simulink model "DA42_Validations"  (Simulink 7.5)
settings: Solver=ode3  StartTime=0.0  StopTime=fdata(end,1)  FixedStep=0.02  RelTol=1e-3
undefined symbols (not defined in the file or in its folder): BHP_A, BHP_B, CP_norm, elebias, fdata, initalt, initbank, initeast, inithead, initnorth, initp, initpitch, initq, initr, initu, initv, initw, mapbias, Pr_Alt, PropEff_norm
libraries: simulink_extras x4, aerolibatmos2 x2
(part 2 of 2)

== system DA42_Validations/DA42/Linear Accelerations and Moments/Cross Prod Moment due to Aero ==
  Vec 1 : Inport
  Vec 2 : Inport  Port=2
  Demux : Demux  Outputs=3
  Demux1 : Demux  Outputs=3
  J axis : Fcn  Expr=u[4]*u[3] - u[6]*u[1]
  Mux : Mux  Inputs=6
  Mux1 : Mux  Inputs=3
  i axis : Fcn  Expr=u[6]*u[2] - u[5]*u[3]
  k axis : Fcn  Expr=u[5]*u[1] - u[4]*u[2]
  X Prod : Outport
  wires:
  Mux1/1 -> X Prod/1
  k axis/1 -> Mux1/3
  i axis/1 -> Mux1/1
  J axis/1 -> Mux1/2
  Mux/1 -> k axis/1, J axis/1, i axis/1
  Demux/2 -> Mux/2
  Demux/3 -> Mux/3
  Demux1/1 -> Mux/4
  Demux1/2 -> Mux/5
  Demux1/3 -> Mux/6
  Demux/1 -> Mux/1
  Vec 1/1 -> Demux/1
  Vec 2/1 -> Demux1/1

== system DA42_Validations/DA42/Linear Accelerations and Moments/Thrust Components ==
  Feng : Inport
  Bus Selector : BusSelector  OutputSignals=L_Thrust,R_Thrust
  Sum : Sum  Inputs=|++
  X Percent : Gain  Gain=0.9669
  Y Percent : Gain  Gain=0
  Z Percent : Gain  Gain=-0.03310
  X% : Outport
  Y% : Outport  Port=2
  Z% : Outport  Port=3
  wires:
  Sum/1 -> Z Percent/1, Y Percent/1, X Percent/1
  Bus Selector/2 -> Sum/2  "<R_Thrust>"
  Bus Selector/1 -> Sum/1  "<L_Thrust>"
  Feng/1 -> Bus Selector/1
  Z Percent/1 -> Z%/1
  Y Percent/1 -> Y%/1
  X Percent/1 -> X%/1

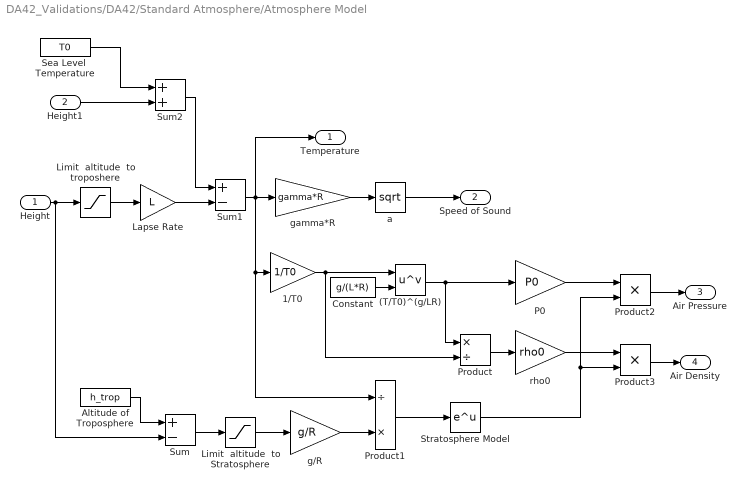
== system DA42_Validations/DA42/Standard Atmosphere/Atmosphere Model ==
  Height : Inport  OutDataType=sfix(16)  OutScaling=2^0
  Height1 : Inport  Port=2  OutDataType=sfix(16)  OutScaling=2^0
  "(T/T0)^(g/LR) " : Math  Operator=pow  OutDataType=sfix(16)  OutScaling=2^0  SaturateOnIntegerOverflow=on
  1/T0 : Gain  Gain=1/T0  ParameterDataType=sfix(16)  ParameterScaling=2^0  OutDataType=sfix(16)  OutScaling=2^0  SaturateOnIntegerOverflow=on  OutDataTypeStr=Inherit: Same as input  ParamDataTypeStr=Inherit: Same as input
  Altitude of Troposphere : Constant  Value=h_trop  OutDataType=sfix(16)  OutScaling=2^0  OutDataTypeStr=Inherit: Inherit via back propagation
  Constant : Constant  Value=g/(L*R)  OutDataType=sfix(16)  OutScaling=2^0  OutDataTypeStr=Inherit: Inherit via back propagation
  Lapse Rate : Gain  Gain=L  ParameterDataType=sfix(16)  ParameterScaling=2^0  OutDataType=sfix(16)  OutScaling=2^0  SaturateOnIntegerOverflow=on  OutDataTypeStr=Inherit: Same as input  ParamDataTypeStr=Inherit: Same as input
  Limit  altitude  to Stratosphere : Saturate  UpperLimit=0  LowerLimit=h_trop-h_strat
  Limit  altitude  to troposhere : Saturate  UpperLimit=h_trop  LowerLimit=0
  P0 : Gain  Gain=P0  ParameterDataType=sfix(16)  ParameterScaling=2^0  OutDataType=sfix(16)  OutScaling=2^0  SaturateOnIntegerOverflow=on  OutDataTypeStr=Inherit: Same as input  ParamDataTypeStr=Inherit: Same as input
  Product : Product  Inputs=*/  OutDataType=sfix(16)  OutScaling=2^0  SaturateOnIntegerOverflow=on  InputSameDT=on  OutDataTypeStr=Inherit: Same as first input
  Product1 : Product  Inputs=/*  OutDataType=sfix(16)  OutScaling=2^0  SaturateOnIntegerOverflow=on  InputSameDT=on  OutDataTypeStr=Inherit: Same as first input
  Product2 : Product  OutDataType=sfix(16)  OutScaling=2^0  SaturateOnIntegerOverflow=on  InputSameDT=on  OutDataTypeStr=Inherit: Same as first input
  Product3 : Product  OutDataType=sfix(16)  OutScaling=2^0  SaturateOnIntegerOverflow=on  InputSameDT=on  OutDataTypeStr=Inherit: Same as first input
  Sea Level  Temperature : Constant  Value=T0  OutDataType=sfix(16)  OutScaling=2^0  OutDataTypeStr=Inherit: Inherit via back propagation
  Stratosphere Model : Math  OutDataType=sfix(16)  OutScaling=2^0  SaturateOnIntegerOverflow=on
  Sum : Sum  Inputs=+-  OutDataType=sfix(16)  OutScaling=2^0  SaturateOnIntegerOverflow=on  InputSameDT=on  OutDataTypeStr=Inherit: Same as first input
  Sum1 : Sum  Inputs=+-  OutDataType=sfix(16)  OutScaling=2^0  SaturateOnIntegerOverflow=on  InputSameDT=on  OutDataTypeStr=Inherit: Same as first input
  Sum2 : Sum  OutDataType=sfix(16)  OutScaling=2^0  SaturateOnIntegerOverflow=on  InputSameDT=on  OutDataTypeStr=Inherit: Same as first input
  a : Math  Operator=sqrt  OutDataType=sfix(16)  OutScaling=2^0  SaturateOnIntegerOverflow=on
  g/R : Gain  Gain=g/R  ParameterDataType=sfix(16)  ParameterScaling=2^0  OutDataType=sfix(16)  OutScaling=2^0  SaturateOnIntegerOverflow=on  OutDataTypeStr=Inherit: Same as input  ParamDataTypeStr=Inherit: Same as input
  gamma*R : Gain  Gain=gamma*R  ParameterDataType=sfix(16)  ParameterScaling=2^0  OutDataType=sfix(16)  OutScaling=2^0  SaturateOnIntegerOverflow=on  OutDataTypeStr=Inherit: Same as input  ParamDataTypeStr=Inherit: Same as input
  rho0 : Gain  Gain=rho0  ParameterDataType=sfix(16)  ParameterScaling=2^0  OutDataType=sfix(16)  OutScaling=2^0  SaturateOnIntegerOverflow=on  OutDataTypeStr=Inherit: Same as input  ParamDataTypeStr=Inherit: Same as input
  Temperature : Outport  OutDataType=sfix(16)  OutScaling=2^0
  Speed of Sound : Outport  Port=2  OutDataType=sfix(16)  OutScaling=2^0
  Air Pressure : Outport  Port=3  OutDataType=sfix(16)  OutScaling=2^0
  Air Density : Outport  Port=4  OutDataType=sfix(16)  OutScaling=2^0
  wires:
  Constant/1 -> "(T/T0)^(g/LR) "/2
  Height/1 -> Limit  altitude  to troposhere/1, Sum/2
  Limit  altitude  to troposhere/1 -> Lapse Rate/1
  Product/1 -> rho0/1
  "(T/T0)^(g/LR) "/1 -> Product/1, P0/1
  1/T0/1 -> "(T/T0)^(g/LR) "/1, Product/2
  gamma*R/1 -> a/1
  a/1 -> Speed of Sound/1
  Sum1/1 -> Temperature/1, gamma*R/1, 1/T0/1, Product1/1
  Lapse Rate/1 -> Sum1/2
  P0/1 -> Product2/1
  Product2/1 -> Air Pressure/1
  rho0/1 -> Product3/1
  Product3/1 -> Air Density/1
  Stratosphere Model/1 -> Product2/2, Product3/2
  g/R/1 -> Product1/2
  Product1/1 -> Stratosphere Model/1
  Altitude of Troposphere/1 -> Sum/1
  Sum/1 -> Limit  altitude  to Stratosphere/1
  Limit  altitude  to Stratosphere/1 -> g/R/1
  Sea Level  Temperature/1 -> Sum2/1
  Sum2/1 -> Sum1/1
  Height1/1 -> Sum2/2

== system DA42_Validations/PowerPlant/Lycoming IO-1/Prop Efficiency  with Cp input ==
  TAS : Inport
  RPS : Inport  Port=2
  Prop D : Inport  Port=3
  CP table : Constant  Value=CP_norm
  Eff vs J : Lookup2D  RowIndex=PropEff_norm(:,1)  ColumnIndex=pitch_Angles  Table=PropEff_norm(:,2:7)  LookUpMeth=Interpolation-Use End Values
  Embedded MATLAB Function Retrieving Pich Angle : Stateflow chart  TreatAsAtomicUnit=on
  J : Fcn  Expr=u(1)/(u(2)*u(3))
  Mux3 : Mux  Inputs=3
  n : Outport
  wires:
  Mux3/1 -> J/1
  [Cp_right] -> Embedded MATLAB Function Retrieving Pich Angle/1(CP)
  Eff vs J/1 -> n/1
  Embedded MATLAB Function Retrieving Pich Angle/1(Pitch) -> Eff vs J/2
  CP table/1 -> Embedded MATLAB Function Retrieving Pich Angle/3(CP_norm)
  J/1 -> Embedded MATLAB Function Retrieving Pich Angle/2(j), Eff vs J/1
  TAS/1 -> Mux3/1
  RPS/1 -> Mux3/2
  Prop D/1 -> Mux3/3

== system DA42_Validations/PowerPlant/Lycoming IO-1/Subsystem ==
  Map : Inport
  RPM1 : Inport  Port=2
  Pressure alt : Inport  Port=3
  Inlet temp C : Inport  Port=4
  15% loss1 : Gain  Gain=.90
  BHP-E : Fcn  Expr=u(1)*sqrt((460+u(2))/(460+u(3)))
  Calculate Cp : Fcn  Expr=550*u(2)/( u(3)*u(4)^3*u(1)^5 )
  L360 Engine  Performance Data : Subsystem
  Mux1 : Mux
  Propellor Diameter (ft) : Constant  Value=6.1667
  "RPM to RPS " : Gain  Gain=1/60
  Cp : Outport
  tag scope: BHP_E_right=global, Prop_D_right=global, RPS_right=global
  wires:
  Map/1 -> L360 Engine  Performance Data/1(MAP)
  L360 Engine  Performance Data/1(BHP-D Ts Ta) -> BHP-E/1
  Propellor Diameter (ft)/1 -> Mux1/1, [Prop_D_right]
  Mux1/1 -> Calculate Cp/1
  L360 Engine  Performance Data/2(Air Density (slugs/ft^3)) -> Mux1/3
  L360 Engine  Performance Data/3(RPM1) -> "RPM to RPS "/1
  "RPM to RPS "/1 -> [RPS_right], Mux1/4
  Calculate Cp/1 -> Cp/1
  BHP-E/1 -> [BHP_E_right], 15% loss1/1
  15% loss1/1 -> Mux1/2
  RPM1/1 -> L360 Engine  Performance Data/2(RPM)
  Pressure alt/1 -> L360 Engine  Performance Data/3(Altitude)
  Inlet temp C/1 -> L360 Engine  Performance Data/4(Inlet air temp)

== system DA42_Validations/PowerPlant/Lycoming IO-1/Thrust ==
  TAS : Inport
  BHP E : Inport  Port=2
  n : Inport  Port=3
  10% loss : Gain  Gain=.90
  Convert to Thrust : Fcn  Expr=(550*u(3)*u(2)/u(1))
  Mux2 : Mux  Inputs=3
  "Thrust " : Outport
  wires:
  Mux2/1 -> Convert to Thrust/1
  Convert to Thrust/1 -> "Thrust "/1
  10% loss/1 -> Mux2/2
  TAS/1 -> Mux2/1
  BHP E/1 -> 10% loss/1
  n/1 -> Mux2/3

== system DA42_Validations/PowerPlant/Lycoming IO-360/Prop Efficiency  with Cp input ==
  TAS : Inport
  RPS : Inport  Port=2
  Prop D : Inport  Port=3
  CP table : Constant  Value=CP_norm
  Eff vs J : Lookup2D  RowIndex=PropEff_norm(:,1)  ColumnIndex=pitch_Angles  Table=PropEff_norm(:,2:7)  LookUpMeth=Interpolation-Use End Values
  Embedded MATLAB Function Retrieving Pich Angle : Stateflow chart  TreatAsAtomicUnit=on
  J : Fcn  Expr=u(1)/(u(2)*u(3))
  Mux3 : Mux  Inputs=3
  n : Outport
  wires:
  Prop D/1 -> Mux3/3
  RPS/1 -> Mux3/2
  TAS/1 -> Mux3/1
  J/1 -> Eff vs J/1, Embedded MATLAB Function Retrieving Pich Angle/2(j)
  CP table/1 -> Embedded MATLAB Function Retrieving Pich Angle/3(CP_norm)
  Embedded MATLAB Function Retrieving Pich Angle/1(Pitch) -> Eff vs J/2
  Eff vs J/1 -> n/1
  [Cp_left] -> Embedded MATLAB Function Retrieving Pich Angle/1(CP)
  Mux3/1 -> J/1

== system DA42_Validations/PowerPlant/Lycoming IO-360/Subsystem ==
  Map : Inport
  RPM1 : Inport  Port=2
  Pressure alt : Inport  Port=3
  Inlet temp C : Inport  Port=4
  15% loss1 : Gain  Gain=.90
  BHP-E : Fcn  Expr=u(1)*sqrt((460+u(2))/(460+u(3)))
  Calculate Cp : Fcn  Expr=550*u(2)/( u(3)*u(4)^3*u(1)^5 )
  L360 Engine  Performance Data : Subsystem
  Mux1 : Mux
  Propellor Diameter (ft) : Constant  Value=6.1667
  "RPM to RPS " : Gain  Gain=1/60
  Cp : Outport
  tag scope: BHP_E_left=global, Prop_D_left=global, RPS_left=global
  wires:
  Inlet temp C/1 -> L360 Engine  Performance Data/4(Inlet air temp)
  Pressure alt/1 -> L360 Engine  Performance Data/3(Altitude)
  RPM1/1 -> L360 Engine  Performance Data/2(RPM)
  15% loss1/1 -> Mux1/2
  BHP-E/1 -> 15% loss1/1, [BHP_E_left]
  Calculate Cp/1 -> Cp/1
  "RPM to RPS "/1 -> Mux1/4, [RPS_left]
  L360 Engine  Performance Data/3(RPM1) -> "RPM to RPS "/1
  L360 Engine  Performance Data/2(Air Density (slugs/ft^3)) -> Mux1/3
  Mux1/1 -> Calculate Cp/1
  Propellor Diameter (ft)/1 -> [Prop_D_left], Mux1/1
  L360 Engine  Performance Data/1(BHP-D Ts Ta) -> BHP-E/1
  Map/1 -> L360 Engine  Performance Data/1(MAP)

== system DA42_Validations/PowerPlant/Lycoming IO-360/Thrust ==
  TAS : Inport
  BHP E : Inport  Port=2
  n : Inport  Port=3
  10% loss : Gain  Gain=.90
  Convert to Thrust : Fcn  Expr=(550*u(3)*u(2)/u(1))
  Mux2 : Mux  Inputs=3
  "Thrust " : Outport
  wires:
  n/1 -> Mux2/3
  BHP E/1 -> 10% loss/1
  TAS/1 -> Mux2/1
  10% loss/1 -> Mux2/2
  Convert to Thrust/1 -> "Thrust "/1
  Mux2/1 -> Convert to Thrust/1

== system DA42_Validations/DA42/Aerodynamics/Aero Forces and Moments/Aerodynamic Forces ==
  CD : Inport
  CY : Inport  Port=2
  CL : Inport  Port=3
  State : Inport  Port=4
  dyn(q) : Inport  Port=5
  Body to Wind : Subsystem
  Bus Selector : BusSelector  OutputSignals=alpha,beta
  Gain : Gain  Gain=-1  SaturateOnIntegerOverflow=on  OutDataTypeStr=Inherit: Same as input  ParamDataTypeStr=Inherit: Same as input
  Gain1 : Gain  Gain=-1  SaturateOnIntegerOverflow=on  OutDataTypeStr=Inherit: Same as input  ParamDataTypeStr=Inherit: Same as input
  Gain2 : Gain  Gain=175.3  SaturateOnIntegerOverflow=on  OutDataTypeStr=Inherit: Same as input  ParamDataTypeStr=Inherit: Same as input
  Math Function : Math  Operator=transpose  SaturateOnIntegerOverflow=on
  Mux : Mux  Inputs=3
  Product : Product  SaturateOnIntegerOverflow=on  OutDataTypeStr=Inherit: Same as first input
  Product1 : Product  Multiplication=Matrix(*)  SaturateOnIntegerOverflow=on  OutDataTypeStr=Inherit: Same as first input
  FaeroBody : Outport
  wires:
  Product1/1 -> FaeroBody/1
  Product/1 -> Product1/2
  Math Function/1 -> Product1/1
  Body to Wind/1(Smatrix) -> Math Function/1
  State/1 -> Bus Selector/1
  dyn(q)/1 -> Gain2/1
  CL/1 -> Gain1/1
  CY/1 -> Mux/2
  CD/1 -> Gain/1
  Gain2/1 -> Product/2
  Mux/1 -> Product/1
  Gain1/1 -> Mux/3
  Gain/1 -> Mux/1
  Bus Selector/1 -> Body to Wind/1(Alpha)  "<alpha>"
  Bus Selector/2 -> Body to Wind/2(Beta)  "<beta>"

== system DA42_Validations/DA42/Aerodynamics/Aero Forces and Moments/Aerodynamic Moments ==
  dyn(q) : Inport
  Croll : Inport  Port=2
  CM : Inport  Port=3
  CN : Inport  Port=4
  Mux : Mux  Inputs=2
  Mux1 : Mux  Inputs=2
  Mux2 : Mux  Inputs=2
  Mux3 : Mux  Inputs=3
  Pitch : Fcn  Expr=u[1] * 175.3*4.17* u[2]
  Roll : Fcn  Expr=u[1] * 175.3*44 * u[2]
  Yaw : Fcn  Expr=u[1] * 175.3*44* u[2]
  Maero : Outport
  wires:
  Mux3/1 -> Maero/1
  CN/1 -> Mux2/2
  CM/1 -> Mux1/2
  Croll/1 -> Mux/2
  dyn(q)/1 -> Mux2/1, Mux1/1, Mux/1
  Yaw/1 -> Mux3/3
  Roll/1 -> Mux3/1
  Pitch/1 -> Mux3/2
  Mux2/1 -> Yaw/1
  Mux1/1 -> Pitch/1
  Mux/1 -> Roll/1

== system DA42_Validations/DA42/Equations of motion numerical integration /Kinematic Equiations/2pi Bound ==
  In : Inport
  2pi : Constant  Value=2*pi
  Math Function : Math  Operator=mod  SaturateOnIntegerOverflow=on
  Out : Outport
  wires:
  In/1 -> Math Function/1
  2pi/1 -> Math Function/2
  Math Function/1 -> Out/1

== system DA42_Validations/DA42/Equations of motion numerical integration /Kinematic Equiations/pi Bound ==
  In : Inport
  2pi : Constant  Value=2*pi
  Math Function : Math  Operator=mod  SaturateOnIntegerOverflow=on
  Sum1 : Sum  Inputs=|+-  SaturateOnIntegerOverflow=on  InputSameDT=on  OutDataTypeStr=Inherit: Same as first input
  Sum2 : Sum  Inputs=|++  SaturateOnIntegerOverflow=on  InputSameDT=on  OutDataTypeStr=Inherit: Same as first input
  pi : Constant  Value=pi
  Out : Outport
  wires:
  Math Function/1 -> Sum1/1
  2pi/1 -> Math Function/2
  In/1 -> Sum2/1
  Sum2/1 -> Math Function/1
  pi/1 -> Sum2/2, Sum1/2
  Sum1/1 -> Out/1

== system DA42_Validations/DA42/Equations of motion numerical integration /Kinematic Equiations/pi Bound1 ==
  In : Inport
  2pi : Constant  Value=2*pi
  Math Function : Math  Operator=mod  SaturateOnIntegerOverflow=on
  Sum1 : Sum  Inputs=|+-  SaturateOnIntegerOverflow=on  InputSameDT=on  OutDataTypeStr=Inherit: Same as first input
  Sum2 : Sum  Inputs=|++  SaturateOnIntegerOverflow=on  InputSameDT=on  OutDataTypeStr=Inherit: Same as first input
  pi : Constant  Value=pi
  Out : Outport
  wires:
  Math Function/1 -> Sum1/1
  2pi/1 -> Math Function/2
  In/1 -> Sum2/1
  Sum2/1 -> Math Function/1
  pi/1 -> Sum2/2, Sum1/2
  Sum1/1 -> Out/1

== system DA42_Validations/DA42/Equations of motion numerical integration /Moment Equations/Inertia Coefs ==
  note: Inertia Coefficeents
      | Page 80 Stevens and Lewis
  note: Jx,Jy,Jz,Jxz
  Inertia : Inport
  Mux : Mux  Inputs=9
  c1 : Fcn  Expr=((u[2]-u[3])*u[3] - u[4]^2)/(u[1]*u[3]-u[4]^2)
  c2 : Fcn  Expr=((u[1]-u[2]+u[3])*u[4])/(u[1]*u[3]-u[4]^2)
  c3 : Fcn  Expr=u[3]/(u[1]*u[3]-u[4]^2)
  c4 : Fcn  Expr=u[4]/(u[1]*u[3]-u[4]^2)
  c5 : Fcn  Expr=(u[3]-u[1])/u[2]
  c6 : Fcn  Expr=u[4]/u[2]
  c7 : Fcn  Expr=1/u[2]
  c8 : Fcn  Expr=(u[1]*(u[1]-u[2])+u[4]^2)/(u[1]*u[3]-u[4]^2)
  c9 : Fcn  Expr=u[1]/(u[1]*u[3]-u[4]^2)
  Iner Coef : Outport
  wires:
  Mux/1 -> Iner Coef/1
  c9/1 -> Mux/9
  c8/1 -> Mux/8
  c7/1 -> Mux/7
  c6/1 -> Mux/6
  c5/1 -> Mux/5
  c4/1 -> Mux/4
  c3/1 -> Mux/3
  c2/1 -> Mux/2
  c1/1 -> Mux/1
  Inertia/1 -> c8/1, c9/1, c7/1, c6/1, c5/1, c4/1, c3/1, c2/1, c1/1

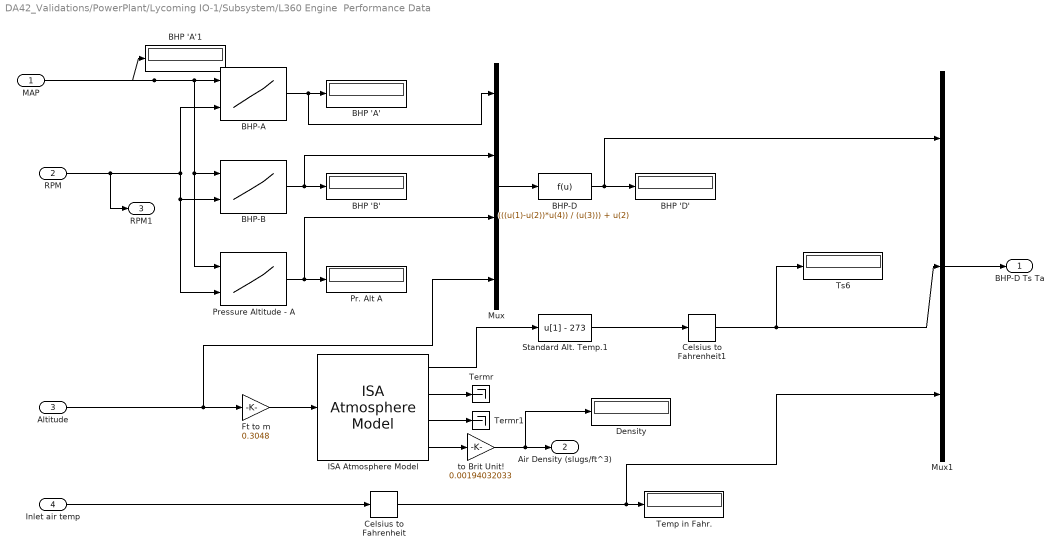
== system DA42_Validations/PowerPlant/Lycoming IO-1/Subsystem/L360 Engine  Performance Data ==
  MAP : Inport
  RPM : Inport  Port=2
  Altitude : Inport  Port=3
  Inlet air temp : Inport  Port=4
  BHP 'A' : Display
  BHP 'A'1 : Display
  BHP 'B' : Display
  BHP 'D' : Display
  BHP-A : Lookup2D  RowIndex=MAP  ColumnIndex=RPM  Table=BHP_A  LookUpMeth=Interpolation-Use End Values
  BHP-B : Lookup2D  RowIndex=MAP  ColumnIndex=RPM  Table=BHP_B  LookUpMeth=Interpolation-Use End Values
  BHP-D : Fcn  Expr=(((u(1)-u(2))*u(4)) / (u(3))) + u(2)
  Celsius to Fahrenheit : simulink_extras/Transformations/Celsius to Fahrenheit  SystemSampleTime=-1
  Celsius to Fahrenheit1 : simulink_extras/Transformations/Celsius to Fahrenheit  SystemSampleTime=-1
  Density : Display
  Ft to m : Gain  Gain=0.3048
  ISA Atmosphere Model : aerolibatmos2/ISA Atmosphere Model  SystemSampleTime=-1  custom=off  g=9.80665  gamma=1.4  R=287.0531  L=0.0065  h_trop=11000  h_strat=20000  rho0=1.225  P0=101325  T0=288.15
  Mux : Mux
  Mux1 : Mux  Inputs=3
  Pr. Alt A : Display
  Pressure Altitude - A : Lookup2D  RowIndex=MAP  ColumnIndex=RPM  Table=Pr_Alt  LookUpMeth=Interpolation-Use End Values
  Standard Alt. Temp.1 : Fcn  Expr=u[1] - 273
  Temp in Fahr. : Display
  Termr : Terminator
  Termr1 : Terminator
  Ts6 : Display
  to Brit Unit! : Gain  Gain=0.00194032033
  BHP-D Ts Ta : Outport
  Air Density (slugs/ft^3) : Outport  Port=2
  RPM1 : Outport  Port=3
  wires:
  RPM/1 -> BHP-A/2, BHP-B/2, Pressure Altitude - A/2, RPM1/1
  BHP-B/1 -> BHP 'B'/1, Mux/2
  BHP-A/1 -> BHP 'A'/1, Mux/1
  Pressure Altitude - A/1 -> Pr. Alt A/1, Mux/3
  Mux/1 -> BHP-D/1
  BHP-D/1 -> BHP 'D'/1, Mux1/1
  Inlet air temp/1 -> Celsius to Fahrenheit/1
  Celsius to Fahrenheit/1 -> Mux1/3, Temp in Fahr./1
  Mux1/1 -> BHP-D Ts Ta/1
  Ft to m/1 -> ISA Atmosphere Model/1
  Standard Alt. Temp.1/1 -> Celsius to Fahrenheit1/1
  Celsius to Fahrenheit1/1 -> Mux1/2, Ts6/1
  ISA Atmosphere Model/2 -> Termr/1
  ISA Atmosphere Model/3 -> Termr1/1
  Altitude/1 -> Mux/4, Ft to m/1
  ISA Atmosphere Model/4 -> to Brit Unit!/1
  to Brit Unit!/1 -> Air Density (slugs/ft^3)/1, Density/1
  ISA Atmosphere Model/1 -> Standard Alt. Temp.1/1
  MAP/1 -> BHP-A/1, BHP-B/1, Pressure Altitude - A/1, BHP 'A'1/1

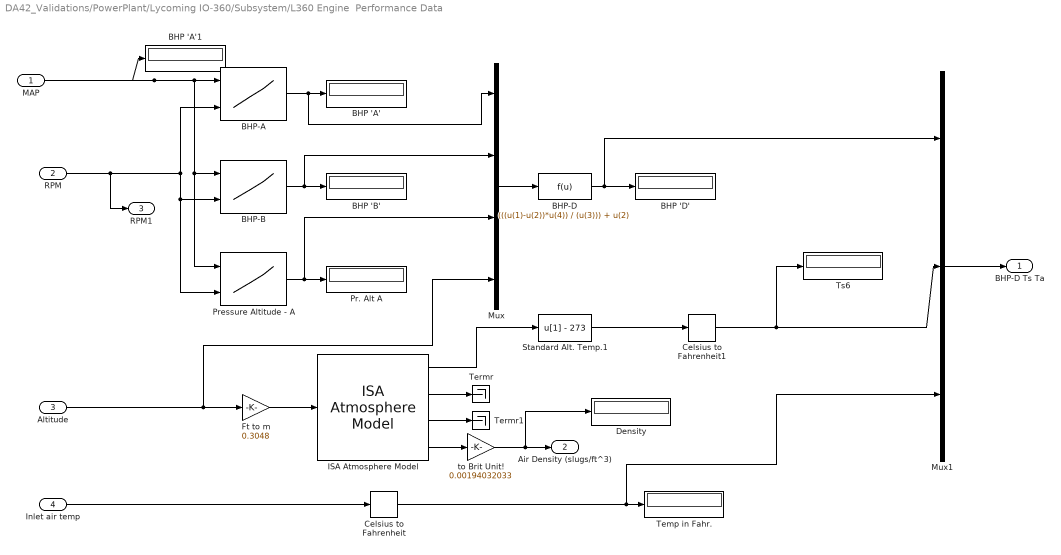
== system DA42_Validations/PowerPlant/Lycoming IO-360/Subsystem/L360 Engine  Performance Data ==
  MAP : Inport
  RPM : Inport  Port=2
  Altitude : Inport  Port=3
  Inlet air temp : Inport  Port=4
  BHP 'A' : Display
  BHP 'A'1 : Display
  BHP 'B' : Display
  BHP 'D' : Display
  BHP-A : Lookup2D  RowIndex=MAP  ColumnIndex=RPM  Table=BHP_A  LookUpMeth=Interpolation-Use End Values
  BHP-B : Lookup2D  RowIndex=MAP  ColumnIndex=RPM  Table=BHP_B  LookUpMeth=Interpolation-Use End Values
  BHP-D : Fcn  Expr=(((u(1)-u(2))*u(4)) / (u(3))) + u(2)
  Celsius to Fahrenheit : simulink_extras/Transformations/Celsius to Fahrenheit  SystemSampleTime=-1
  Celsius to Fahrenheit1 : simulink_extras/Transformations/Celsius to Fahrenheit  SystemSampleTime=-1
  Density : Display
  Ft to m : Gain  Gain=0.3048
  ISA Atmosphere Model : aerolibatmos2/ISA Atmosphere Model  SystemSampleTime=-1  custom=off  g=9.80665  gamma=1.4  R=287.0531  L=0.0065  h_trop=11000  h_strat=20000  rho0=1.225  P0=101325  T0=288.15
  Mux : Mux
  Mux1 : Mux  Inputs=3
  Pr. Alt A : Display
  Pressure Altitude - A : Lookup2D  RowIndex=MAP  ColumnIndex=RPM  Table=Pr_Alt  LookUpMeth=Interpolation-Use End Values
  Standard Alt. Temp.1 : Fcn  Expr=u[1] - 273
  Temp in Fahr. : Display
  Termr : Terminator
  Termr1 : Terminator
  Ts6 : Display
  to Brit Unit! : Gain  Gain=0.00194032033
  BHP-D Ts Ta : Outport
  Air Density (slugs/ft^3) : Outport  Port=2
  RPM1 : Outport  Port=3
  wires:
  MAP/1 -> BHP 'A'1/1, Pressure Altitude - A/1, BHP-B/1, BHP-A/1
  ISA Atmosphere Model/1 -> Standard Alt. Temp.1/1
  to Brit Unit!/1 -> Density/1, Air Density (slugs/ft^3)/1
  ISA Atmosphere Model/4 -> to Brit Unit!/1
  Altitude/1 -> Ft to m/1, Mux/4
  ISA Atmosphere Model/3 -> Termr1/1
  ISA Atmosphere Model/2 -> Termr/1
  Celsius to Fahrenheit1/1 -> Ts6/1, Mux1/2
  Standard Alt. Temp.1/1 -> Celsius to Fahrenheit1/1
  Ft to m/1 -> ISA Atmosphere Model/1
  Mux1/1 -> BHP-D Ts Ta/1
  Celsius to Fahrenheit/1 -> Temp in Fahr./1, Mux1/3
  Inlet air temp/1 -> Celsius to Fahrenheit/1
  BHP-D/1 -> Mux1/1, BHP 'D'/1
  Mux/1 -> BHP-D/1
  Pressure Altitude - A/1 -> Mux/3, Pr. Alt A/1
  BHP-A/1 -> Mux/1, BHP 'A'/1
  BHP-B/1 -> Mux/2, BHP 'B'/1
  RPM/1 -> RPM1/1, Pressure Altitude - A/2, BHP-B/2, BHP-A/2

== system DA42_Validations/DA42/Aerodynamics/Aero Forces and Moments/Aerodynamic Forces/Body to Wind ==
  note: This transforms any arbitrary vector from body axis to wind axis.
      | Page 63  Stevens and Lewis
  Alpha : Inport
  Beta : Inport  Port=2
  -ca sb : Fcn  Expr=-1 * cos(u[1]) * sin(u[2])
  -sa : Fcn  Expr=-1 * sin(u[1])
  -sa sb : Fcn  Expr="-1 * sin(u[1])  * sin(u[2])"
  Fcn8 : Fcn  Expr=cos(u[1])
  Matrix Concatenation : Concatenate  NumInputs=3  Mode=Multidimensional array
  Matrix Concatenation1 : Concatenate  NumInputs=3  Mode=Multidimensional array
  Matrix Concatenation2 : Concatenate  NumInputs=3  Mode=Multidimensional array  ConcatenateDimension=2
  Matrix Concatenation3 : Concatenate  NumInputs=3  Mode=Multidimensional array
  Mux1 : Mux  Inputs=2
  ca cb : Fcn  Expr="cos(u[1]) *  cos(u[2])"
  cb : Fcn  Expr=cos(u[2])
  sa cb : Fcn  Expr=sin(u[1]) * cos(u[2])
  sb : Fcn  Expr=sin(u[2])
  zero : Fcn  Expr=u[1] * 0
  Smatrix : Outport
  wires:
  Matrix Concatenation2/1 -> Smatrix/1
  Beta/1 -> Mux1/2
  Alpha/1 -> Mux1/1
  Mux1/1 -> Fcn8/1, -sa sb/1, sa cb/1, zero/1, cb/1, sb/1, -sa/1, -ca sb/1, ca cb/1
  Fcn8/1 -> Matrix Concatenation3/3
  -sa sb/1 -> Matrix Concatenation3/2
  sa cb/1 -> Matrix Concatenation3/1
  cb/1 -> Matrix Concatenation1/2
  sb/1 -> Matrix Concatenation1/1
  zero/1 -> Matrix Concatenation1/3
  -sa/1 -> Matrix Concatenation/3
  ca cb/1 -> Matrix Concatenation/1
  -ca sb/1 -> Matrix Concatenation/2
  Matrix Concatenation3/1 -> Matrix Concatenation2/3
  Matrix Concatenation1/1 -> Matrix Concatenation2/2
  Matrix Concatenation/1 -> Matrix Concatenation2/1

== matlab function PowerPlant/Lycoming IO-360/Prop Efficiency with Cp input/Embedded MATLAB Function Retrieving Pich Angle ==
  data: CP input double; j input double; CP_norm input double; Pitch output double
function Pitch   =  fcn(CP, j, CP_norm)
%#eml

proppitch= [15 20 25 30 35 40];
tempJ = 0;
tempCP = 0;
Jindex = 1;
CPindex = 1;
% j = 0.4;
% CP = 0.22;

i=0;
for i=1:size(CP_norm,1)
    if j > CP_norm(i,1)
        
        tempJ = CP_norm(i,1);
        Jindex = i;
    end
end
for a=1:size(CP_norm,2)
    if CP > CP_norm(Jindex,a)
        tempCP = CP_norm(a,1);
        CPindex = a;
    end
end

if (CPindex ~= 0 && Jindex ~= 0)
    if (CPindex) == 7;
        Pitch = 40 ; 
    else
        if CPindex == 1
            Pitch =15;
        else
            Pitch = interp1(CP_norm(Jindex,CPindex:CPindex+1),proppitch(CPindex-1:CPindex),CP);
        end
        
    end
else
    Pitch = 15;

end
return

== matlab function PowerPlant/Lycoming IO-1/Prop Efficiency with Cp input/Embedded MATLAB Function Retrieving Pich Angle ==
  data: CP input double; j input double; CP_norm input double; Pitch output double
function Pitch   =  fcn(CP, j, CP_norm)
%#eml

proppitch= [15 20 25 30 35 40];
tempJ = 0;
tempCP = 0;
Jindex = 1;
CPindex = 1;
% j = 0.4;
% CP = 0.22;

i=0;
for i=1:size(CP_norm,1)
    if j > CP_norm(i,1)
        
        tempJ = CP_norm(i,1);
        Jindex = i;
    end
end
for a=1:size(CP_norm,2)
    if CP > CP_norm(Jindex,a)
        tempCP = CP_norm(a,1);
        CPindex = a;
    end
end

if (CPindex ~= 0 && Jindex ~= 0)
    if (CPindex) == 7;
        Pitch = 40 ; 
    else
        if CPindex == 1
            Pitch =15;
        else
            Pitch = interp1(CP_norm(Jindex,CPindex:CPindex+1),proppitch(CPindex-1:CPindex),CP);
        end
        
    end
else
    Pitch = 15;

end
return
